simulink model "PID"  (R2018a)
settings: Solver=VariableStepAuto  StartTime=0.0  StopTime=10.0  RelTol=1e-3
settings Model: Creator=mattclark  LastModifiedBy=mattclark
settings SFSimCC: SimCustomHeaderCode="#include \"driver.h\""  SimUserSources=driver.c

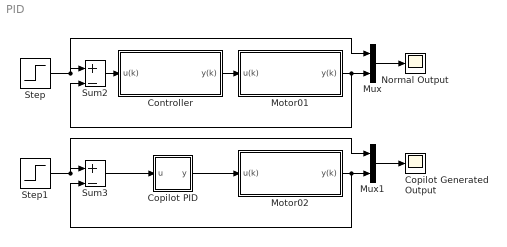
== system PID ==
  Controller : Subsystem
  Copilot Generated Output : Scope
  Copilot PID : MATLAB Function  TreatAsAtomicUnit=on
  Motor01 : Subsystem
  Motor02 : Subsystem
  Mux : Mux  Inputs=2
  Mux1 : Mux  Inputs=2
  Normal Output : Scope
  Step : Step  Time=.2  SampleTime=0
  Step1 : Step  Time=.2  SampleTime=0
  Sum2 : Sum  Inputs=|+-
  Sum3 : Sum  Inputs=|+-
  wires:
  Step/1 -> Mux/1, Sum2/1
  Motor01/1(y(k)) -> Sum2/2, Mux/2
  Controller/1(y(k)) -> Motor01/1(u(k))
  Mux/1 -> Normal Output/1
  Sum2/1 -> Controller/1(u(k))
  Step1/1 -> Mux1/1, Sum3/1
  Copilot PID/1(y) -> Motor02/1(u(k))
  Sum3/1 -> Copilot PID/1(u)
  Mux1/1 -> Copilot Generated Output/1
  Motor02/1(y(k)) -> Sum3/2, Mux1/2

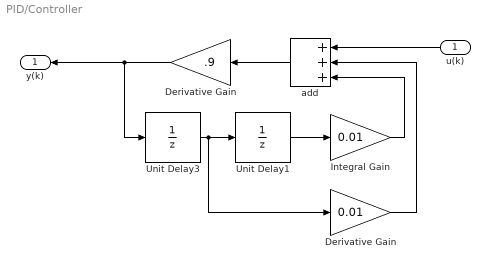
== system PID/Controller ==
  u(k) : Inport
  Derivative Gain : Gain  Gain=0.01
  "Derivative Gain " : Gain  Gain=.9
  "Integral Gain " : Gain  Gain=0.01
  Unit Delay1 : UnitDelay  SampleTime=-1
  Unit Delay3 : UnitDelay  SampleTime=-1
  add : Sum  Inputs=+++
  y(k) : Outport
  wires:
  add/1 -> "Derivative Gain "/1
  Unit Delay3/1 -> Derivative Gain/1, Unit Delay1/1
  u(k)/1 -> add/1
  "Derivative Gain "/1 -> y(k)/1, Unit Delay3/1
  "Integral Gain "/1 -> add/3
  Unit Delay1/1 -> "Integral Gain "/1
  Derivative Gain/1 -> add/2

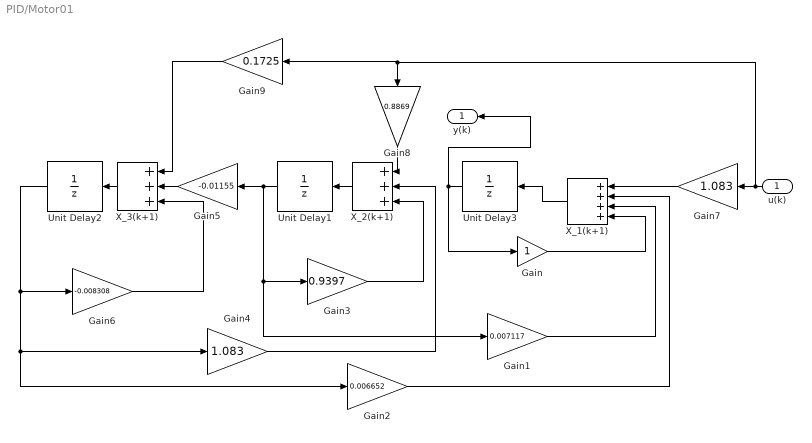
== system PID/Motor01 ==
  u(k) : Inport
  Gain : Gain
  Gain1 : Gain  Gain=0.007117
  Gain2 : Gain  Gain=0.006652
  Gain3 : Gain  Gain=0.9397
  Gain4 : Gain  Gain=1.083
  Gain5 : Gain  Gain=-0.01155
  Gain6 : Gain  Gain=-0.008308
  Gain7 : Gain  Gain=1.083
  Gain8 : Gain  Gain=0.8869
  Gain9 : Gain  Gain=0.1725
  Unit Delay1 : UnitDelay  SampleTime=-1
  Unit Delay2 : UnitDelay  SampleTime=-1
  Unit Delay3 : UnitDelay  SampleTime=-1
  X_1(k+1) : Sum  Inputs=++++
  X_2(k+1) : Sum  Inputs=+++
  X_3(k+1) : Sum  Inputs=+++
  y(k) : Outport
  wires:
  X_3(k+1)/1 -> Unit Delay2/1
  X_1(k+1)/1 -> Unit Delay3/1
  X_2(k+1)/1 -> Unit Delay1/1
  Unit Delay3/1 -> y(k)/1, Gain/1
  Gain/1 -> X_1(k+1)/4
  Unit Delay1/1 -> Gain5/1, Gain1/1, Gain3/1
  Gain1/1 -> X_1(k+1)/3
  Unit Delay2/1 -> Gain4/1, Gain2/1, Gain6/1
  Gain2/1 -> X_1(k+1)/2
  Gain3/1 -> X_2(k+1)/3
  Gain4/1 -> X_2(k+1)/2
  Gain5/1 -> X_3(k+1)/2
  Gain6/1 -> X_3(k+1)/3
  Gain7/1 -> X_1(k+1)/1
  u(k)/1 -> Gain8/1, Gain9/1, Gain7/1
  Gain8/1 -> X_2(k+1)/1
  Gain9/1 -> X_3(k+1)/1

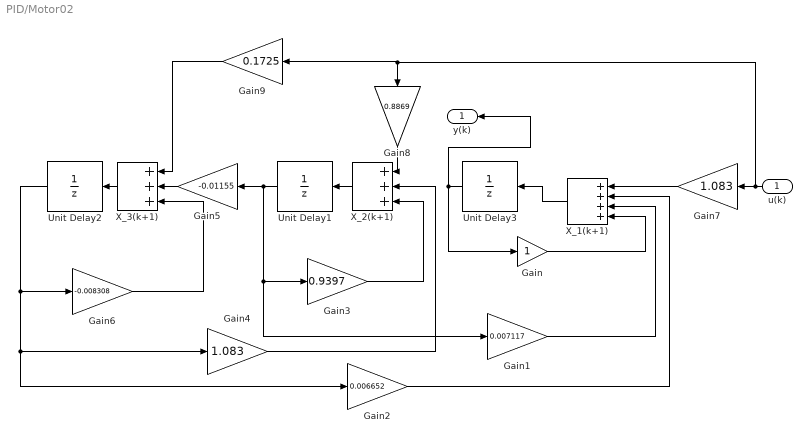
== system PID/Motor02 ==
  u(k) : Inport
  Gain : Gain
  Gain1 : Gain  Gain=0.007117
  Gain2 : Gain  Gain=0.006652
  Gain3 : Gain  Gain=0.9397
  Gain4 : Gain  Gain=1.083
  Gain5 : Gain  Gain=-0.01155
  Gain6 : Gain  Gain=-0.008308
  Gain7 : Gain  Gain=1.083
  Gain8 : Gain  Gain=0.8869
  Gain9 : Gain  Gain=0.1725
  Unit Delay1 : UnitDelay  SampleTime=-1
  Unit Delay2 : UnitDelay  SampleTime=-1
  Unit Delay3 : UnitDelay  SampleTime=-1
  X_1(k+1) : Sum  Inputs=++++
  X_2(k+1) : Sum  Inputs=+++
  X_3(k+1) : Sum  Inputs=+++
  y(k) : Outport
  wires:
  X_3(k+1)/1 -> Unit Delay2/1
  X_1(k+1)/1 -> Unit Delay3/1
  X_2(k+1)/1 -> Unit Delay1/1
  Unit Delay3/1 -> y(k)/1, Gain/1
  Gain/1 -> X_1(k+1)/4
  Unit Delay1/1 -> Gain5/1, Gain1/1, Gain3/1
  Gain1/1 -> X_1(k+1)/3
  Unit Delay2/1 -> Gain4/1, Gain2/1, Gain6/1
  Gain2/1 -> X_1(k+1)/2
  Gain3/1 -> X_2(k+1)/3
  Gain4/1 -> X_2(k+1)/2
  Gain5/1 -> X_3(k+1)/2
  Gain6/1 -> X_3(k+1)/3
  Gain7/1 -> X_1(k+1)/1
  u(k)/1 -> Gain8/1, Gain9/1, Gain7/1
  Gain8/1 -> X_2(k+1)/1
  Gain9/1 -> X_3(k+1)/1

== matlab function PID/Copilot PID ==
  data: u input; y output
function y = driver(u)
y = 0.0;
y = coder.ceval('driver',u);
